simulink model "ParentsPhone"  (R2023a)
settings: Solver=FixedStepAuto  StartTime=0.0  StopTime=inf  RelTol=1e-3
libraries: androidaudiovideolib x4, androidcommunicationlib x4, androiduilib x2
settings Model: Creator=ketha  LastModifiedBy=ketha
settings OptimizationCC: EnhancedBackFolding=on  PassReuseOutputArgsAs=Individual arguments  ZeroExternalMemoryAtStartup=off  ZeroInternalMemoryAtStartup=off  MaxStackSize=64  OptimizeBlockOrder=speed  DifferentSizesBufferReuse=on  OptimizationCustomize=off  EfficientTunableParamExpr=on
settings DebuggingCC: ParameterTunabilityLossMsg=error
settings HardwareCC: ProdBitPerPointer=32  ProdBitPerSizeT=32  ProdBitPerPtrDiffT=32  ProdLargestAtomicInteger=Long  ProdLargestAtomicFloat=Double  ProdWordSize=32  ProdHWDeviceType=ARM Compatible->ARM Cortex
settings SFSimCC: MATLABDynamicMemAlloc=off
settings RTWCC: Description=Embedded Coder  SystemTargetFile=ert.tlc  HardwareBoard=Android Device  TLCOptions="-aInlineSetEventsForThisBaseRateFcn=TLC_FALSE -aSuppressMultiTaskScheduler=TLC_FALSE  -aRateBasedStepFcn=0"  TemplateMakefile=ert_default_tmf  RTWVerbose=off  Toolchain=Android SDK/NDK Tools
settings CodeAppCC: ForceParamTrailComments=on  IgnoreCustomStorageClasses=off  OperatorAnnotations=on  SimulinkDataObjDesc=on  SFDataObjDesc=on  InsertBlockDesc=on

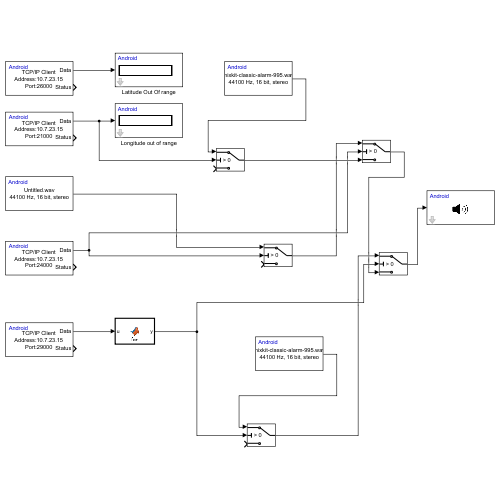
[thumbnail: Simulink's stored preview of the top-level diagram]
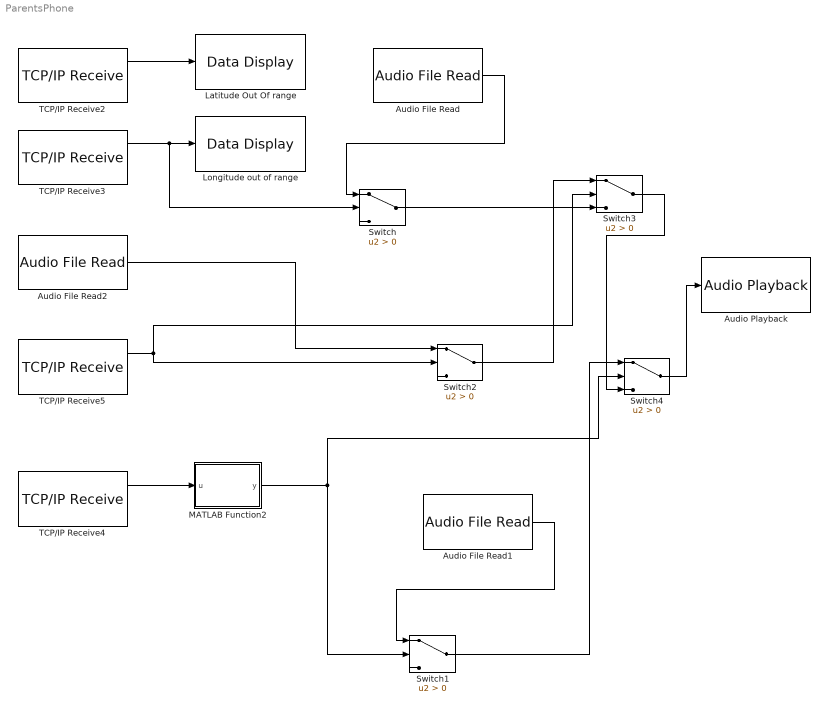
== system ParentsPhone ==
  Audio File Read : androidaudiovideolib/Audio File Read  FileName=C:\Users\ketha\OneDrive\Desktop\Darshan_c\Darshan_SSRP\mixkit-classic-alarm-995.wav  FrameSize=4410
  Audio File Read1 : androidaudiovideolib/Audio File Read  FileName=C:\Users\ketha\OneDrive\Desktop\Darshan_c\Darshan_SSRP\mixkit-classic-alarm-995.wav  FrameSize=4410
  Audio File Read2 : androidaudiovideolib/Audio File Read  FileName=C:\Users\ketha\OneDrive\Desktop\Darshan_c\Darshan_SSRP\Untitled.wav  FrameSize=4410
  Audio Playback : androidaudiovideolib/Audio Playback  SampleFreq=44100  AudioSamplingFreq=44100  SampleTime=0.1  DeviceStr=0  QueueDuration=0  BlockPlatform=Android
  Latitude Out Of range : androiduilib/Data Display  DataDisplayId=ParentsPhone/Latitude_Out_Of_range  Format=Float  Precision=6  SimulateUsing=Code generation  blockPlatform=Android
  Longitude out of range : androiduilib/Data Display  DataDisplayId=ParentsPhone/Longitude_out_of_range  Format=Float  Precision=6  SimulateUsing=Code generation  blockPlatform=Android
  MATLAB Function2 : MATLAB Function  TreatAsAtomicUnit=on
  Switch{,1..4} (5 alike) : Switch  Criteria=u2 > Threshold  SaturateOnIntegerOverflow=off  InputSameDT=off
  TCP/IP Receive2 : androidcommunicationlib/TCP//IP Receive  TCPReceiveId=ParentsPhone/TCP//IP_Receive2  Mode_=Client  LocalServerPort_=25000  RemoteAddr_=10.7.23.15  RemoteServerPort_=26000  DataType_=int16  DataSize_=1  SampleTime_=0.1  ClientPortBindingSelection_=off  ClientPortToBind_=35000  BlockingMode_=off  BlockTimeout_=0.1
  TCP/IP Receive3 : androidcommunicationlib/TCP//IP Receive  TCPReceiveId=ParentsPhone/TCP//IP_Receive3  Mode_=Client  LocalServerPort_=25000  RemoteAddr_=10.7.23.15  RemoteServerPort_=21000  DataType_=int16  DataSize_=1  SampleTime_=0.1  ClientPortBindingSelection_=off  ClientPortToBind_=35000  BlockingMode_=off  BlockTimeout_=0.1
  TCP/IP Receive4 : androidcommunicationlib/TCP//IP Receive  TCPReceiveId=ParentsPhone/TCP//IP_Receive4  Mode_=Client  LocalServerPort_=25000  RemoteAddr_=10.7.23.15  RemoteServerPort_=29000  DataType_=int16  DataSize_=1  SampleTime_=0.1  ClientPortBindingSelection_=off  ClientPortToBind_=35000  BlockingMode_=off  BlockTimeout_=0.1
  TCP/IP Receive5 : androidcommunicationlib/TCP//IP Receive  TCPReceiveId=ParentsPhone/TCP//IP_Receive5  Mode_=Client  LocalServerPort_=25000  RemoteAddr_=10.7.23.15  RemoteServerPort_=24000  DataType_=int16  DataSize_=1  SampleTime_=0.1  ClientPortBindingSelection_=off  ClientPortToBind_=35000  BlockingMode_=off  BlockTimeout_=0.1
  wires:
  Audio File Read/1 -> Switch/1
  TCP/IP Receive2/1 -> Latitude Out Of range/1
  TCP/IP Receive3/1 -> Switch/2, Longitude out of range/1
  Switch/1 -> Switch3/3
  Switch4/1 -> Audio Playback/1
  TCP/IP Receive4/1 -> MATLAB Function2/1(u)
  MATLAB Function2/1(y) -> Switch1/2, Switch4/2
  Audio File Read1/1 -> Switch1/1
  Switch1/1 -> Switch4/1
  Audio File Read2/1 -> Switch2/1
  Switch2/1 -> Switch3/1
  Switch3/1 -> Switch4/3
  TCP/IP Receive5/1 -> Switch3/2, Switch2/2

== matlab function ParentsPhone/MATLAB Function2 ==
  data: u input; y output
function y = fcn(u)

% Specify y as single data type
y = single(u);

if u > 10
    y = single(1); % Use single() to specify the data type
else
    y = single(0); % Use single() to specify the data type
end
